simulink model "IBVS_me_model_4_13_2025"  (R2023b)
settings: Solver=FixedStepDiscrete  StartTime=0.0  StopTime=5  FixedStep=.001  MaxStep=0.005  RelTol=1e-3
values from neighbouring files (symbols this model uses):
  dT = 1/frequency    (= 0.005)    [init_IBVS_me_4_13_2025.m]
  init_pose = [C ; ang']    [init_IBVS_me_4_13_2025.m]
  initial_Config = Config*pi/180    [init_IBVS_me_4_13_2025.m]
  Kd = 5*eye(4)    [init_IBVS_me_4_13_2025.m]
  Kp = 10*eye(4)    [init_IBVS_me_4_13_2025.m]
  p1 = [0.34; -.65; .035]    [init_IBVS_me_4_13_2025.m]
  p2 = [0.44; -.64; .035]    [init_IBVS_me_4_13_2025.m]
  ref = [ref1; ref2]    [init_IBVS_me_4_13_2025.m]
undefined symbols (not defined in the file or in its folder): f, O
libraries: robotmaniplib x3, simulink x1, matrix_library x1, vrlib x1
settings Model: Creator=Acer  LastModifiedBy=admin
settings SolverCC: AlgebraicLoopSolver=TrustRegion
settings DebuggingCC: UnconnectedInputMsg=warning  UnconnectedOutputMsg=warning  UnconnectedLineMsg=warning
settings ModelReferenceCC: EnableRefExpFcnMdlSchedulingChecks=on
settings RTWCC: DLArmComputeVersion=19.05

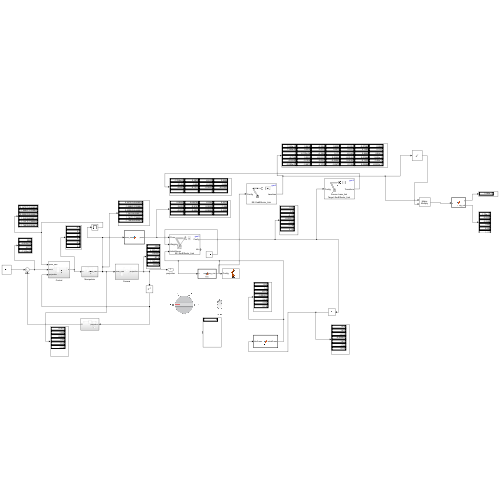
[thumbnail: Simulink's stored preview of the top-level diagram]
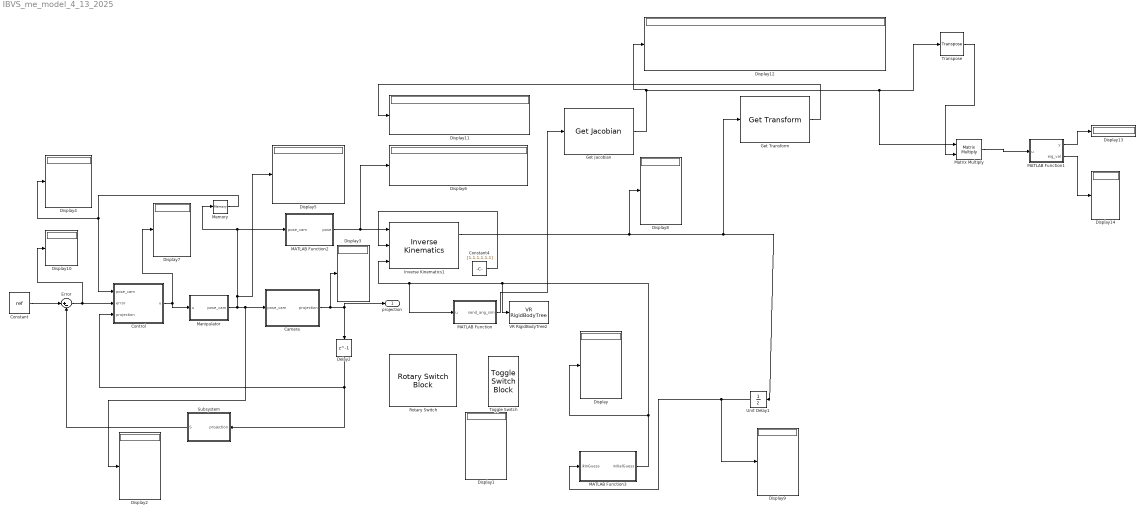
== system IBVS_me_model_4_13_2025 ==
  Camera : Subsystem
  Constant : Constant  Value=ref  SampleTime=-1
  Constant4 : Constant  Value=[1,1,1,1,1,1]
  Control : Subsystem
  Delay2 : Delay  DelayLength=1  InitialCondition=[536.47 ; 447.23 ;1;763.4880;505.5745;1]
  Display{,1..14} (15 alike) : Display
  Error : Sum  Inputs=|+-
  Get Jacobian : robotmaniplib/Get Jacobian  RigidBodyTree=gen3  EndEffector=EndEffector_Link  SimulateUsing=Interpreted execution
  Get Transform : robotmaniplib/Get Transform  RigidBodyTree=gen3  SourceBody=base_link  TargetBody=EndEffector_Link  SimulateUsing=Interpreted execution
  Inverse Kinematics1 : robotmaniplib/Inverse Kinematics  RigidBodyTree=gen3  EndEffector=EndEffector_Link  ShowInfo=on  SolverName=BFGS Gradient Projection  EnforceJointLimits=off  MaxIterations=1500  MaxTime=10  GradientTolerance=1e-7  SolutionTolerance=1e-5  StepTolerance=1e-14  ErrorChangeTolerance=1e-12  UseErrorDamping=on  DampingBias=0.0025  SimulateUsing=Interpreted execution
  MATLAB Function : MATLAB Function  TreatAsAtomicUnit=on
  MATLAB Function1 : MATLAB Function  TreatAsAtomicUnit=on
  MATLAB Function2 : MATLAB Function  TreatAsAtomicUnit=on
  MATLAB Function3 : MATLAB Function  TreatAsAtomicUnit=on
  Manipulator : Subsystem
  Matrix Multiply : Product  Multiplication=Matrix(*)
  Memory : Memory  InitialCondition=init_pose
  Rotary Switch : RotarySwitchBlock  LabelPosition=Bottom
      settings: Values={{'Off', 'Low', 'Medium', 'High'}, [0 0.1 0.2 0.3]}
  Subsystem : Subsystem
  Toggle Switch : ToggleSwitchBlock  LabelPosition=Bottom
      settings: Values={{'Off', 'On'}, [0 1]}
  Transpose : matrix_library/Transpose
  Unit Delay1 : UnitDelay  InitialCondition=initial_Config  SampleTime=-1  HasFrameUpgradeWarning=on
  VR RigidBodyTree2 : vrlib/VR RigidBodyTree  RBT=gen3  useRBT=on  Ts=-1  ForceViewerOpen=on
  projection : Outport
  wires:
  Camera/1(projection) -> Display3/1, projection/1, Delay2/1
  Delay2/1 -> Control/3(projection), Subsystem/1(projection)
  Memory/1 -> Control/1(pose_cam), Display4/1
  Control/1(u) -> Manipulator/1(u), Display7/1
  Error/1 -> Display10/1, Control/2(error)
  Manipulator/1(pose_cam) -> Display5/1, Memory/1, MATLAB Function2/1(pose_cam), Display2/1, Camera/1(pose_cam)
  Constant/1 -> Error/1
  Subsystem/1(S) -> Error/2
  MATLAB Function2/1(pose) -> Display6/1, Inverse Kinematics1/1
  Constant4/1 -> Inverse Kinematics1/2
  MATLAB Function3/1(initialGuess) -> VR RigidBodyTree2/1, MATLAB Function/1(u), Inverse Kinematics1/3, Display/1
  Unit Delay1/1 -> Display9/1, MATLAB Function3/1(ikInGuess)
  Inverse Kinematics1/1 -> Get Transform/1, Unit Delay1/1, Display8/1
  MATLAB Function/1(send_ang_sim) -> Get Jacobian/1
  Get Transform/1 -> Display11/1
  Get Jacobian/1 -> Matrix Multiply/1, Transpose/1, Display12/1
  Matrix Multiply/1 -> MATLAB Function1/1(u)
  MATLAB Function1/1(y) -> Display13/1
  Transpose/1 -> Matrix Multiply/2
  MATLAB Function1/2(eig_val) -> Display14/1

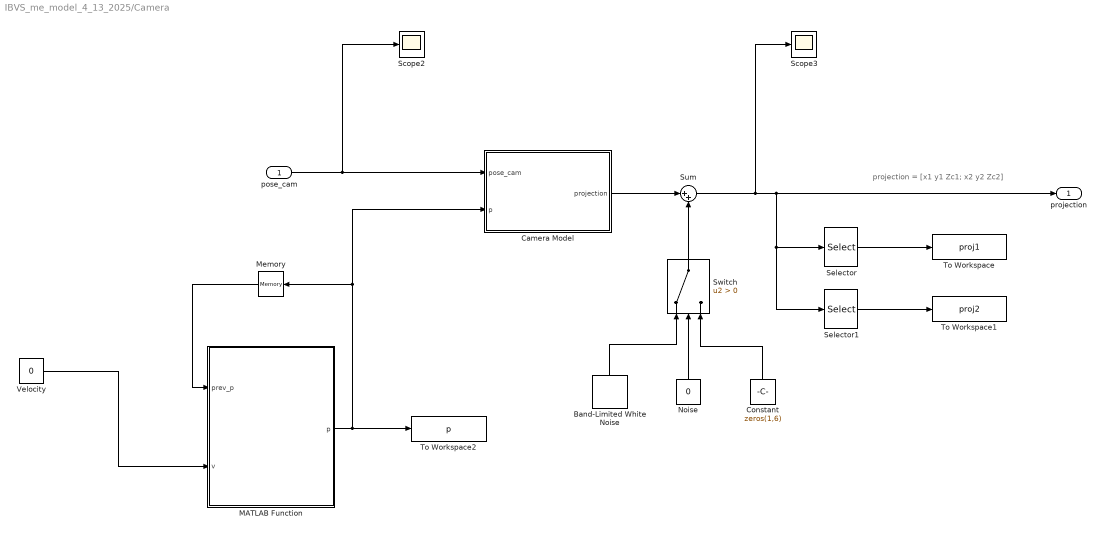
== system IBVS_me_model_4_13_2025/Camera ==
  note: projection = [x1 y1 Zc1; x2 y2 Zc2]
  pose_cam : Inport
  Band-Limited White Noise : simulink/Sources/Band-Limited White Noise  Cov=[0.00001 0.00001 0.00001 0.00001 0.00001 0.00001]  Ts=0.01  seed=[23341 10 14 19 2123 186]
  Camera Model : MATLAB Function  TreatAsAtomicUnit=on
  Constant : Constant  Value=zeros(1,6)
  MATLAB Function : MATLAB Function  TreatAsAtomicUnit=on  SystemSampleTime=dT
  Memory : Memory  InitialCondition=[p1; p2]
  Noise : Constant  Value=0
  Scope2 : Scope
  Scope3 : Scope
  Selector : Selector  InputPortWidth=6  IndexOptions=Index vector (dialog)  Indices=[1 2]  OutputSizes=1
  Selector1 : Selector  InputPortWidth=6  IndexOptions=Index vector (dialog)  Indices=[4 5]  OutputSizes=1
  Sum : Sum  Inputs=|++
  Switch : Switch  Criteria=u2 > Threshold  SaturateOnIntegerOverflow=off  InputSameDT=off
  To Workspace : ToWorkspace  VariableName=proj1  SampleTime=0.1
  To Workspace1 : ToWorkspace  VariableName=proj2  SampleTime=0.1
  To Workspace2 : ToWorkspace  VariableName=p  SampleTime=0.1
  Velocity : Constant  Value=0  SampleTime=dT
  projection : Outport
  wires:
  pose_cam/1 -> Scope2/1, Camera Model/1(pose_cam)
  Selector1/1 -> To Workspace1/1
  Selector/1 -> To Workspace/1
  Camera Model/1(projection) -> Sum/1
  Sum/1 -> Scope3/1, projection/1, Selector1/1, Selector/1
  Switch/1 -> Sum/2
  Noise/1 -> Switch/2
  Band-Limited White Noise/1 -> Switch/1
  Constant/1 -> Switch/3
  MATLAB Function/1(p) -> Camera Model/2(p), Memory/1, To Workspace2/1
  Memory/1 -> MATLAB Function/1(prev_p)
  Velocity/1 -> MATLAB Function/2(v)

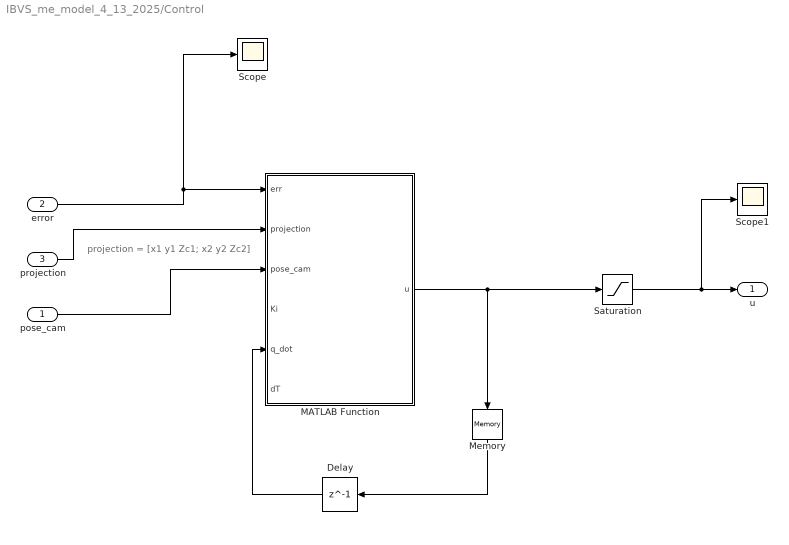
== system IBVS_me_model_4_13_2025/Control ==
  note: projection = [x1 y1 Zc1; x2 y2 Zc2]
  pose_cam : Inport
  error : Inport  Port=2
  projection : Inport  Port=3
  Delay : Delay  DelayLength=1
  MATLAB Function : MATLAB Function  TreatAsAtomicUnit=on  SystemSampleTime=1/200
  Memory : Memory  InitialCondition=zeros(6,1)
  Saturation : Saturate
  Scope : Scope
  Scope1 : Scope
  u : Outport
  wires:
  error/1 -> Scope/1, MATLAB Function/1(err)
  pose_cam/1 -> MATLAB Function/3(pose_cam)
  Delay/1 -> MATLAB Function/5(q_dot)
  Memory/1 -> Delay/1
  projection/1 -> MATLAB Function/2(projection)
  MATLAB Function/1(u) -> Saturation/1, Memory/1
  Saturation/1 -> Scope1/1, u/1

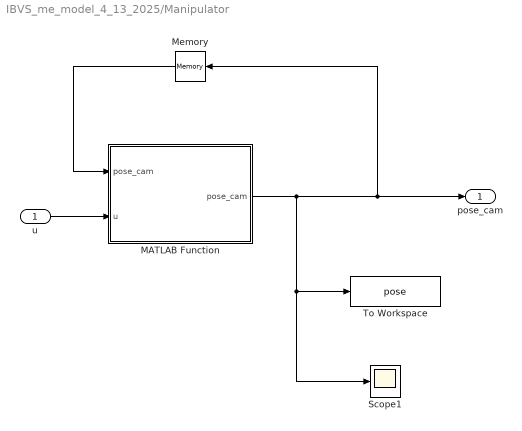
== system IBVS_me_model_4_13_2025/Manipulator ==
  u : Inport
  MATLAB Function : MATLAB Function  TreatAsAtomicUnit=on  SystemSampleTime=1/200
  Memory : Memory  InitialCondition=init_pose
  Scope1 : Scope
  To Workspace : ToWorkspace  VariableName=pose  SampleTime=0.1
  pose_cam : Outport
  wires:
  u/1 -> MATLAB Function/2(u)
  Memory/1 -> MATLAB Function/1("pose_cam ")
  MATLAB Function/1(pose_cam) -> Scope1/1, To Workspace/1, Memory/1, pose_cam/1

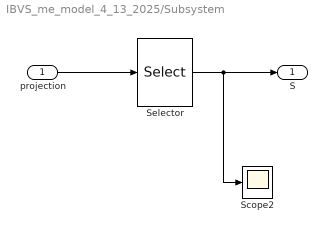
== system IBVS_me_model_4_13_2025/Subsystem ==
  projection : Inport
  Scope2 : Scope
  Selector : Selector  InputPortWidth=6  IndexOptions=Index vector (dialog)  Indices=[1 2 4 5]  OutputSizes=1
  S : Outport
  wires:
  projection/1 -> Selector/1
  Selector/1 -> Scope2/1, S/1

== matlab function IBVS_me_model_4_13_2025/Control/MATLAB Function ==
  data: err input; projection input; pose_cam input; Kp parameter; u output; p2 parameter; Kd parameter; Ki input; q_dot input; p1 parameter; dT input
function u = fcn(err, projection, pose_cam, Kp, p2, Kd,Ki, q_dot, p1,dT)

% projection = [x1 y1 Zc1; x2 y2 Zc2]
x1 = projection(1);         % x projection in the image plane
y1 = projection(2);         % y projection
Zc1 = projection(3);
x2 = projection(4);
y2 = projection(5);
Zc2 = projection(6);
ang = pose_cam(4:6);  % camera's orientation 

if Zc1 == 0 || isnan(Zc1)
    Zc1 = p1(3)- pose_cam(3);
end

if Zc2 == 0 || isnan(Zc2)
    Zc2 = p2(3) - pose_cam(3);
end

% Interaction matrix (feature to Camera?)
Ls1 = [ -1/Zc1     0     x1/Zc1     x1*y1    -(1+x1^2)     y1;  
        0       -1/Zc1   y1/Zc1    1+y1^2      -x1*y1     -x1];
    
Ls2 = [ -1/Zc2     0     x2/Zc2     x2*y2    -(1+x2^2)     y2;  
        0       -1/Zc2   y2/Zc2    1+y2^2      -x2*y2     -x2];
    
Ls = [Ls1; Ls2];

% Trasformation (Camera to base rotation?)
Rx = [1   0       0   ;
      0 cos(ang(1)) -sin(ang(1));
      0 sin(ang(1)) cos(ang(1))];

Ry = [cos(ang(2)) 0 sin(ang(2)) ;
       0     1   0    ;
     -sin(ang(2)) 0 cos(ang(2))];
 
Rz = [cos(ang(3)) -sin(ang(3)) 0;
      sin(ang(3))  cos(ang(3)) 0;
       0      0     1];

Rc = Rz * Ry * Rx;

%Camera to base angular velocity transofrmation - rate of change of euler angles = J2*[wx wy
%wz} and rate of change of euler angles*J2^-1 = [wx wy wz]
J2 = [1     sin(ang(1))*tan(ang(2))    cos(ang(1))*tan(ang(2));
      0           cos(ang(1))                  -sin(ang(1));
      0     sin(ang(1))/cos(ang(2))    cos(ang(1))/cos(ang(2)) ];

J = eye(6);  % Jacobian J(q)


%[Rc' zeros(3); zeros(3) J2^-1]*q_dot where q_dot(1:3) is linear velosity
%and q_dot(4:6) is angular velocity so Rc gets multiplied by q_dot(1:3) and
%J2 inverse by q_dot(4:6)
Jl = Ls * [Rc' zeros(3); zeros(3) J2^-1] * J;

%q_dot has rate of change of euler angles, ie linear and angular motion
%spevcified in world frame? which gets transported to feature frame.
%inverse of jl will transport the thing in bracket ie.  (Kp * err - Kd * Jl
%* q_dot) from feature frame to world frame
% IBVS control Law
pose_cam
u = pinv(Jl) * (Kp * err + Kd * Jl * q_dot + Ki*err*dT)

== matlab function IBVS_me_model_4_13_2025/Camera/Camera Model ==
  data: projection output; f parameter; O parameter; pose_cam input; p input
function projection = proj(f, O, pose_cam, p)

d = pose_cam(1:3) - O;    % camera's position in world frame
ang = pose_cam(4:6);      % camera's orientation 
p1 = p(1:3);
p2 = p(4:6);

%%
Rx = [1   0       0   ;
      0 cos(ang(1)) -sin(ang(1));
      0 sin(ang(1)) cos(ang(1))];

Ry = [cos(ang(2)) 0 sin(ang(2)) ;
       0     1   0    ;
     -sin(ang(2)) 0 cos(ang(2))];
 
Rz = [cos(ang(3)) -sin(ang(3)) 0;
      sin(ang(3))  cos(ang(3)) 0;
       0      0     1];


Rc = Rz * Ry * Rx;


Twc = [Rc            d;
      zeros(1,3)     1];

%%
%P = diag([f(1),f(2),1]) * [eye(3), zeros(3,1)]; % camera projection matrix, assumes that the image is centered at (0,0)
P = [f(1) 0 640.3222 0;0, f(2),237.1297 0;0 0 1 0];

p_cam1 = Twc^-1 * [p1; 1];   % point's position in camera frame
p_cam2 = Twc^-1 * [p2; 1];

p_tilde1 = P * p_cam1;
p_tilde2 = P * p_cam2;

x_proj1 = p_tilde1(1)/p_cam1(3);
y_proj1 = p_tilde1(2)/p_cam1(3);
Zc1 = p_cam1(3);

x_proj2 = p_tilde2(1)/p_cam2(3);
y_proj2 = p_tilde2(2)/p_cam2(3);
Zc2 = p_cam2(3);


projection  = [x_proj1; y_proj1; Zc1; x_proj2; y_proj2; Zc2]; %; x_proj2; y_proj2; Zc2];

end

== matlab function IBVS_me_model_4_13_2025/Manipulator/MATLAB Function ==
  data: pose_cam input; u input; pose_cam output; dT parameter
function pose_cam = fcn(pose_cam,u, dT)

position = zeros(3, 1);
angle = zeros(3, 1);
%ang = u(4:6)
ang=pose_cam(4:6)

Rx = [1   0       0   ;
      0 cos(ang(1)) -sin(ang(1));
      0 sin(ang(1)) cos(ang(1))];

Ry = [cos(ang(2)) 0 sin(ang(2)) ;
       0     1   0    ;
     -sin(ang(2)) 0 cos(ang(2))];
 
Rz = [cos(ang(3)) -sin(ang(3)) 0;
      sin(ang(3))  cos(ang(3)) 0;
       0      0     1];

J1 = Rz * Ry * Rx; %rc from world to camera frame, u is the linear velocity

J2 = [1     sin(ang(1))*tan(ang(2))    cos(ang(1))*tan(ang(2));
      0           cos(ang(1))                  -sin(ang(1));
      0     sin(ang(1))/cos(ang(2))    cos(ang(1))/cos(ang(2)) ];


position = pose_cam(1:3) + J1 * u(1:3) * dT
%angle = pose_cam(4:6) + J2 * ang * dT
angle = pose_cam(4:6) + J2 * u(4:6) * dT
pose_cam = [position; angle];

== matlab function IBVS_me_model_4_13_2025/Camera/MATLAB Function ==
  data: prev_p input; p output; v input; dT parameter
function p = fcn(prev_p ,v, dT)

p1 = prev_p(1:3);
p2 = prev_p(4:6);

p1 = p1 + [0; v; 0] * dT;
p2 = p2 + [0; v; 0] * dT;

p = [p1; p2];

== matlab function IBVS_me_model_4_13_2025/MATLAB Function ==
  data: u input; send_ang_sim output
function send_ang_sim = fcn(u)
%#codegen
send_ang_sim=wrapTo2Pi(u)

== matlab function IBVS_me_model_4_13_2025/MATLAB Function1 ==
  data: u input; y output; eig_val output
function [y,eig_val] = fcn(u)
y=det(u);
eig_val=eig(u);

== matlab function IBVS_me_model_4_13_2025/MATLAB Function2 ==
  data: pose_cam input; pose output
function pose = fcn(pose_cam)

pose = trvec2tform(pose_cam(1:3)') * eul2tform(pose_cam(4:6)');

== matlab function IBVS_me_model_4_13_2025/MATLAB Function3 ==
  data: ikInGuess input; initialGuess output
function initialGuess = fcn(ikInGuess)

initialGuess = wrapToPi(ikInGuess)
%initialGuess=ikInGuess
